simulink model "beam_control_ic_tx"  (R2022b)
settings: Solver=FixedStepAuto  StartTime=0.0  StopTime=100e-7  RelTol=1e-3
values from neighbouring files (symbols this model uses):
  beam_former_gain_array = [1 1]    [beam_control_ic_tx_parameter.m]
  Bias = 0    [ModelingRFSystemsWithAntennaArraysUsingAntennaBlockExample.m]    (also in beam_control_ic_rx_parameter.m)
  filter_gain0_0 = 0    [ModelingRFSystemsWithAntennaArraysUsingAntennaBlockExample.m]    (also in beam_control_ic_rx_parameter.m)
  filter_gain0_1 = 1/6    (= 0.166666666667)    [ModelingRFSystemsWithAntennaArraysUsingAntennaBlockExample.m]    (also in beam_control_ic_rx_parameter.m)
  filter_gain0_2 = 2/3    (= 0.666666666667)    [ModelingRFSystemsWithAntennaArraysUsingAntennaBlockExample.m]    (also in beam_control_ic_rx_parameter.m)
  filter_gain0_3 = 1/6    (= 0.166666666667)    [ModelingRFSystemsWithAntennaArraysUsingAntennaBlockExample.m]    (also in beam_control_ic_rx_parameter.m)
  filter_gain1_0 = 0    [ModelingRFSystemsWithAntennaArraysUsingAntennaBlockExample.m]    (also in beam_control_ic_rx_parameter.m)
  filter_gain1_1 = 1/2    (= 0.5)    [ModelingRFSystemsWithAntennaArraysUsingAntennaBlockExample.m]    (also in beam_control_ic_rx_parameter.m)
  filter_gain1_2 = 0    [ModelingRFSystemsWithAntennaArraysUsingAntennaBlockExample.m]    (also in beam_control_ic_rx_parameter.m)
  filter_gain1_3 = -1/2    (= -0.5)    [ModelingRFSystemsWithAntennaArraysUsingAntennaBlockExample.m]    (also in beam_control_ic_rx_parameter.m)
  filter_gain2_0 = 0    [ModelingRFSystemsWithAntennaArraysUsingAntennaBlockExample.m]    (also in beam_control_ic_rx_parameter.m)
  filter_gain2_1 = 1/2    (= 0.5)    [ModelingRFSystemsWithAntennaArraysUsingAntennaBlockExample.m]    (also in beam_control_ic_rx_parameter.m)
  filter_gain2_2 = -1    [ModelingRFSystemsWithAntennaArraysUsingAntennaBlockExample.m]    (also in beam_control_ic_rx_parameter.m)
  filter_gain2_3 = 1/2    (= 0.5)    [ModelingRFSystemsWithAntennaArraysUsingAntennaBlockExample.m]    (also in beam_control_ic_rx_parameter.m)
  filter_gain3_0 = 1/6    (= 0.166666666667)    [ModelingRFSystemsWithAntennaArraysUsingAntennaBlockExample.m]    (also in beam_control_ic_rx_parameter.m)
  filter_gain3_1 = -1/2    (= -0.5)    [ModelingRFSystemsWithAntennaArraysUsingAntennaBlockExample.m]    (also in beam_control_ic_rx_parameter.m)
  filter_gain3_2 = 1/2    (= 0.5)    [ModelingRFSystemsWithAntennaArraysUsingAntennaBlockExample.m]    (also in beam_control_ic_rx_parameter.m)
  filter_gain3_3 = -1/6    (= -0.166666666667)    [ModelingRFSystemsWithAntennaArraysUsingAntennaBlockExample.m]    (also in beam_control_ic_rx_parameter.m)
  fraction_delay = 1.5    [ModelingRFSystemsWithAntennaArraysUsingAntennaBlockExample.m]    (also in beam_control_ic_rx_parameter.m = 1)
  integer_delay = 0    [ModelingRFSystemsWithAntennaArraysUsingAntennaBlockExample.m]    (also in beam_control_ic_rx_parameter.m)
  N = 10    [ModelingRFSystemsWithAntennaArraysUsingAntennaBlockExample.m]    (also in beam_control_ic_rx_parameter.m)
  Ref = 2.048    [ModelingRFSystemsWithAntennaArraysUsingAntennaBlockExample.m]    (also in beam_control_ic_rx_parameter.m)
undefined symbols (not defined in the file or in its folder): fdesignblkfcn, gcbh, pskmod
libraries: dspsigops x5, simulink_extras x2, msbDacArchitectures x2, dspmlti4 x2, commrfcorlib x2, commeq3 x2
(part 1 of 2)
settings Model: Creator=BOBO  LastModifiedBy=BOBO

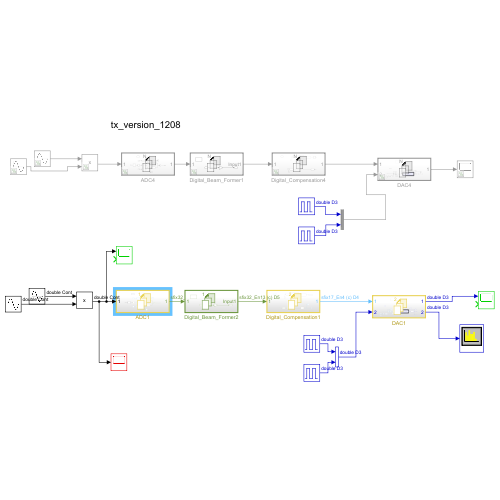
[thumbnail: Simulink's stored preview of the top-level diagram]
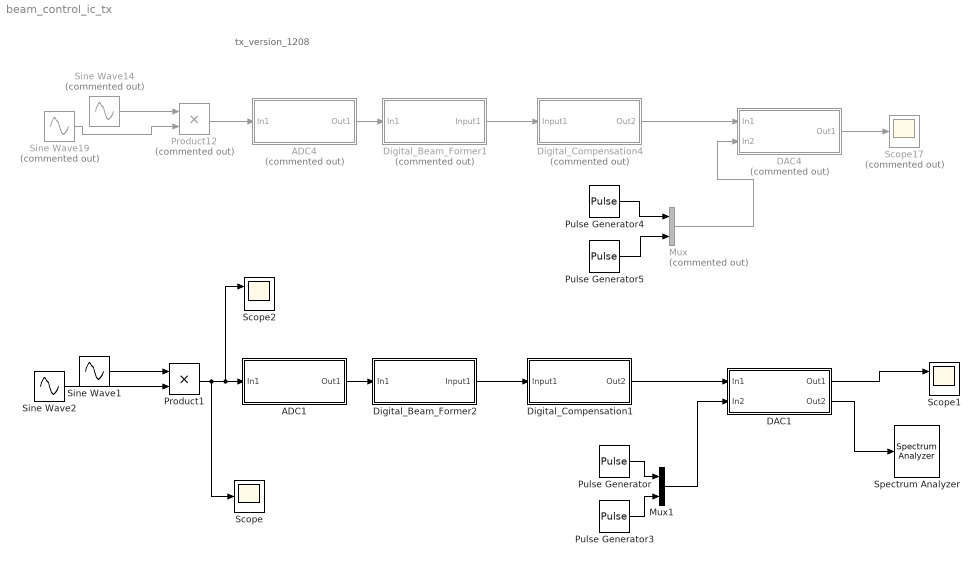
== system beam_control_ic_tx ==
  note: tx_version_1208
  ADC1 : Subsystem  TreatAsAtomicUnit=on
  ADC4 : Subsystem  Commented=on  TreatAsAtomicUnit=on
  DAC1 : Subsystem  TreatAsAtomicUnit=on
  DAC4 : Subsystem  Commented=on  TreatAsAtomicUnit=on
  Digital_Beam_Former1 : Subsystem  Commented=on  TreatAsAtomicUnit=on
  Digital_Beam_Former2 : Subsystem  TreatAsAtomicUnit=on
  Digital_Compensation1 : Subsystem  TreatAsAtomicUnit=on
  Digital_Compensation4 : Subsystem  Commented=on  TreatAsAtomicUnit=on
  Mux : Mux  Commented=on  Inputs=2
  Mux1 : Mux  Inputs=2
  Product1 : Product
  Product12 : Product  Commented=on
  Pulse Generator{,3..5} (4 alike) : DiscretePulseGenerator  PulseType=Time based  Period=1e-9  PulseWidth=50
  Scope : Scope
  Scope1 : Scope  NumInputPorts=2
  Scope17 : Scope  Commented=on
  Scope2 : Scope  NumInputPorts=2
  Sine Wave1 : Sin  Frequency=2*pi*3.25e9  SampleTime=0
  Sine Wave14 : Sin  Commented=on  Frequency=2*pi*3.25e9  SampleTime=0
  Sine Wave19 : Sin  Commented=on  Frequency=2*pi*62.5e6  SampleTime=0
  Sine Wave2 : Sin  Frequency=2*pi*62.5e6  SampleTime=0
  Spectrum Analyzer : SpectrumAnalyzer
  wires:
  Digital_Compensation4/1(Out2) -> DAC4/1(In1)
  ADC4/1(Out1) -> Digital_Beam_Former1/1(In1)
  Sine Wave14/1 -> Product12/1
  Sine Wave19/1 -> Product12/2
  Product12/1 -> ADC4/1(In1)
  DAC4/1(Out1) -> Scope17/1
  Digital_Beam_Former1/1(Input1) -> Digital_Compensation4/1(Input1)
  Pulse Generator4/1 -> Mux/1
  Pulse Generator5/1 -> Mux/2
  Mux/1 -> DAC4/2(In2)
  Mux1/1 -> DAC1/2(In2)
  Pulse Generator3/1 -> Mux1/2
  Pulse Generator/1 -> Mux1/1
  Digital_Beam_Former2/1(Input1) -> Digital_Compensation1/1(Input1)
  Product1/1 -> Scope/1, Scope2/1, ADC1/1(In1)
  Sine Wave2/1 -> Product1/2
  Sine Wave1/1 -> Product1/1
  ADC1/1(Out1) -> Digital_Beam_Former2/1(In1)
  Digital_Compensation1/1(Out2) -> DAC1/1(In1)
  DAC1/2(Out2) -> Spectrum Analyzer/1
  DAC1/1(Out1) -> Scope1/1

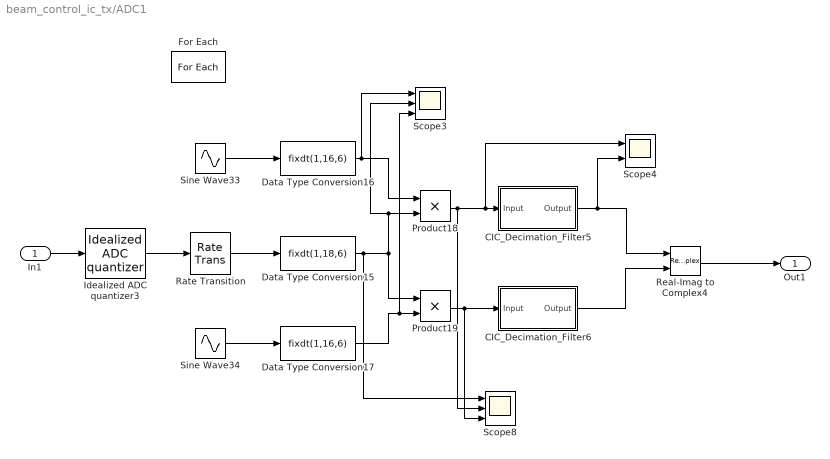
== system beam_control_ic_tx/ADC1 ==
  In1 : Inport  Partition=on  PartitionDimension=1  PartitionWidth=1  PartitionOffset=0
  CIC_Decimation_Filter5 : Subsystem  Tag=FilterWizardSubSystem
      settings: ErrorFcn=dspFilterRealizedInBasicElemsAlgLoopErrFcnCallback
  CIC_Decimation_Filter6 : Subsystem  Tag=FilterWizardSubSystem
      settings: ErrorFcn=dspFilterRealizedInBasicElemsAlgLoopErrFcnCallback
  Data Type Conversion15 : DataTypeConversion  OutDataTypeStr=fixdt(1,18,6)  SaturateOnIntegerOverflow=off  RndMeth=Floor
  Data Type Conversion16 : DataTypeConversion  OutDataTypeStr=fixdt(1,16,6)  SaturateOnIntegerOverflow=off  RndMeth=Floor
  Data Type Conversion17 : DataTypeConversion  OutDataTypeStr=fixdt(1,16,6)  SaturateOnIntegerOverflow=off  RndMeth=Floor
  For Each : ForEach  DisableCoverage=on
  Idealized ADC quantizer3 : simulink_extras/Additional Discrete/Idealized ADC quantizer  NumberOfConverterBits=8  Vmin=-1  Vmax=1  OutputDataType=double  OutputNegativeValues=on
  Product18 : Product
  Product19 : Product
  Rate Transition : RateTransition  OutPortSampleTime=1/1e9
  Real-Imag to Complex4 : RealImagToComplex
  Scope3 : Scope  NumInputPorts=3
  Scope4 : Scope  NumInputPorts=2
  Scope8 : Scope  NumInputPorts=3
  Sine Wave33 : Sin  Frequency=2*pi*250e6  Phase=1.57  SampleTime=1/1e9
  Sine Wave34 : Sin  Frequency=2*pi*250e6  SampleTime=1/1e9
  Out1 : Outport  ConcatenationDimension=1
  wires:
  CIC_Decimation_Filter6/1(Output) -> Real-Imag to Complex4/2
  Sine Wave33/1 -> Data Type Conversion16/1
  Product19/1 -> CIC_Decimation_Filter6/1(Input), Scope8/3
  Data Type Conversion16/1 -> Scope3/1, Product18/1
  Sine Wave34/1 -> Data Type Conversion17/1
  Data Type Conversion17/1 -> Product19/2, Scope3/3
  Real-Imag to Complex4/1 -> Out1/1
  In1/1 -> Idealized ADC quantizer3/1
  Rate Transition/1 -> Data Type Conversion15/1
  Idealized ADC quantizer3/1 -> Rate Transition/1
  Data Type Conversion15/1 -> Scope3/2, Product18/2, Product19/1, Scope8/1
  Product18/1 -> Scope8/2, CIC_Decimation_Filter5/1(Input), Scope4/1
  CIC_Decimation_Filter5/1(Output) -> Real-Imag to Complex4/1, Scope4/2

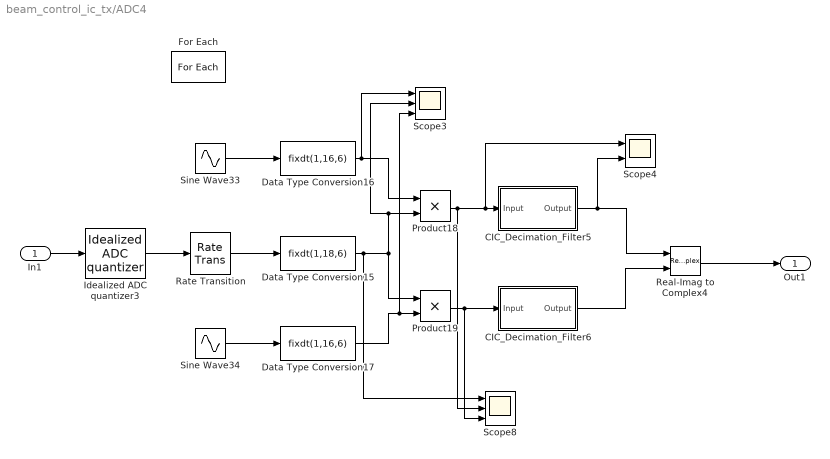
== system beam_control_ic_tx/ADC4 ==
  In1 : Inport  Partition=on  PartitionDimension=1  PartitionWidth=1  PartitionOffset=0
  CIC_Decimation_Filter5 : Subsystem  Tag=FilterWizardSubSystem
      settings: ErrorFcn=dspFilterRealizedInBasicElemsAlgLoopErrFcnCallback
  CIC_Decimation_Filter6 : Subsystem  Tag=FilterWizardSubSystem
      settings: ErrorFcn=dspFilterRealizedInBasicElemsAlgLoopErrFcnCallback
  Data Type Conversion15 : DataTypeConversion  OutDataTypeStr=fixdt(1,18,6)  SaturateOnIntegerOverflow=off  RndMeth=Floor
  Data Type Conversion16 : DataTypeConversion  OutDataTypeStr=fixdt(1,16,6)  SaturateOnIntegerOverflow=off  RndMeth=Floor
  Data Type Conversion17 : DataTypeConversion  OutDataTypeStr=fixdt(1,16,6)  SaturateOnIntegerOverflow=off  RndMeth=Floor
  For Each : ForEach  DisableCoverage=on
  Idealized ADC quantizer3 : simulink_extras/Additional Discrete/Idealized ADC quantizer  NumberOfConverterBits=12  Vmin=-1  Vmax=1  OutputDataType=double  OutputNegativeValues=on
  Product18 : Product
  Product19 : Product
  Rate Transition : RateTransition  OutPortSampleTime=1/1e9
  Real-Imag to Complex4 : RealImagToComplex
  Scope3 : Scope  NumInputPorts=3
  Scope4 : Scope  NumInputPorts=2
  Scope8 : Scope  NumInputPorts=3
  Sine Wave33 : Sin  Frequency=2*pi*250e6  Phase=1.57  SampleTime=1/1e9
  Sine Wave34 : Sin  Frequency=2*pi*250e6  SampleTime=1/1e9
  Out1 : Outport  ConcatenationDimension=1
  wires:
  CIC_Decimation_Filter5/1(Output) -> Scope4/2, Real-Imag to Complex4/1
  Product18/1 -> Scope4/1, CIC_Decimation_Filter5/1(Input), Scope8/2
  Data Type Conversion15/1 -> Scope8/1, Product19/1, Product18/2, Scope3/2
  Idealized ADC quantizer3/1 -> Rate Transition/1
  Rate Transition/1 -> Data Type Conversion15/1
  In1/1 -> Idealized ADC quantizer3/1
  Real-Imag to Complex4/1 -> Out1/1
  Data Type Conversion17/1 -> Scope3/3, Product19/2
  Sine Wave34/1 -> Data Type Conversion17/1
  Data Type Conversion16/1 -> Product18/1, Scope3/1
  Product19/1 -> Scope8/3, CIC_Decimation_Filter6/1(Input)
  Sine Wave33/1 -> Data Type Conversion16/1
  CIC_Decimation_Filter6/1(Output) -> Real-Imag to Complex4/2

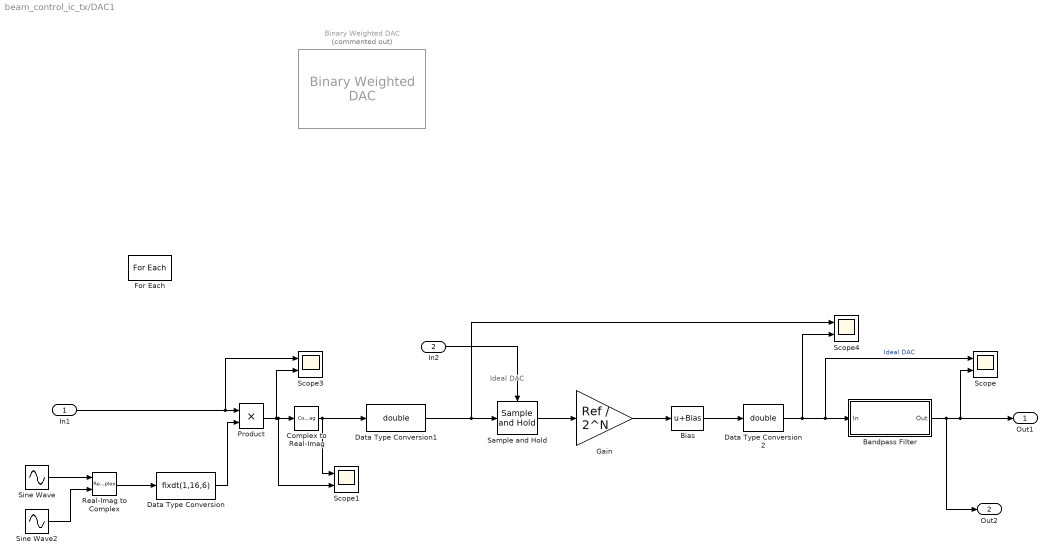
== system beam_control_ic_tx/DAC1 ==
  note: Ideal DAC
  In1 : Inport  Partition=on  PartitionDimension=1  PartitionWidth=1  PartitionOffset=0
  In2 : Inport  Port=2  Partition=on  PartitionDimension=1  PartitionWidth=1  PartitionOffset=0
  Bandpass Filter : Subsystem  DialogController=fdesignblkfcn  InitFcn=fdesignblkfcn(gcbh, {'InitFcn'});  mask(Bandpass Filter){}
      mask help: Design a bandpass filter
      settings: CopyFcn=fdesignblkfcn(gcbh, {'CopyFcn'});
      mask Help: helpview(mapfilelocation('dsp'), 'dspbandpassfilter');
      mask Display: disp('Bandpass');
  Bias : Bias  Bias=Bias  SaturateOnIntegerOverflow=off
  Binary Weighted DAC : msbDacArchitectures/Binary Weighted DAC  Commented=on  NBits=5  Polarity=Bipolar  ExtStartClk=on  StartFreq=1e6  Ref=2  Bias=0  ReadySignal=off  EnableLinearityImpairments=on  OffsetError=0  OffsetErrorUnit=LSB  GainError=0  GainErrorUnit=LSB  EnableTimingImpairments=on  TimingSpecification=Settling time  SettlingTime=2e-7  SettlingTimeTolerance=0.5  RisingSlewRate=5015625  FallingSlewRate=-5015625
  Complex to Real-Imag : ComplexToRealImag  Output=Real
  Data Type Conversion : DataTypeConversion  OutDataTypeStr=fixdt(1,16,6)  SaturateOnIntegerOverflow=off  RndMeth=Floor
  Data Type Conversion1 : DataTypeConversion  OutDataTypeStr=double  SaturateOnIntegerOverflow=off  RndMeth=Floor
  Data Type Conversion2 : DataTypeConversion  OutDataTypeStr=double  SaturateOnIntegerOverflow=off  RndMeth=Floor
  For Each : ForEach  DisableCoverage=on
  Gain : Gain  Gain=Ref / 2^N
  Product : Product
  Real-Imag to Complex : RealImagToComplex
  Sample and Hold : dspsigops/Sample and Hold  trig=Rising edge  initCond=0  latchinput=off
  Scope{,1,3..4} (4 alike) : Scope  NumInputPorts=2
  Sine Wave : Sin  Frequency=2*pi*250e6  Phase=1.57  SampleTime=1/1e9
  Sine Wave2 : Sin  Frequency=2*pi*250e6  SampleTime=1/1e9
  Out1 : Outport  ConcatenationDimension=1
  Out2 : Outport  Port=2  ConcatenationDimension=1
  wires:
  Bandpass Filter/1(Out) -> Out2/1, Out1/1, Scope/2
  In2/1 -> Sample and Hold/Trigger
  Sample and Hold/1 -> Gain/1
  Gain/1 -> Bias/1
  Bias/1 -> Data Type Conversion2/1
  Data Type Conversion1/1 -> Sample and Hold/1, Scope4/1
  Data Type Conversion2/1 -> Bandpass Filter/1(In), Scope/1, Scope4/2  "Ideal DAC"
  Real-Imag to Complex/1 -> Data Type Conversion/1
  Sine Wave2/1 -> Real-Imag to Complex/2
  Sine Wave/1 -> Real-Imag to Complex/1
  In1/1 -> Scope3/1, Product/1
  Product/1 -> Scope3/2, Complex to Real-Imag/1, Scope1/2
  Complex to Real-Imag/1 -> Scope1/1, Data Type Conversion1/1
  Data Type Conversion/1 -> Product/2

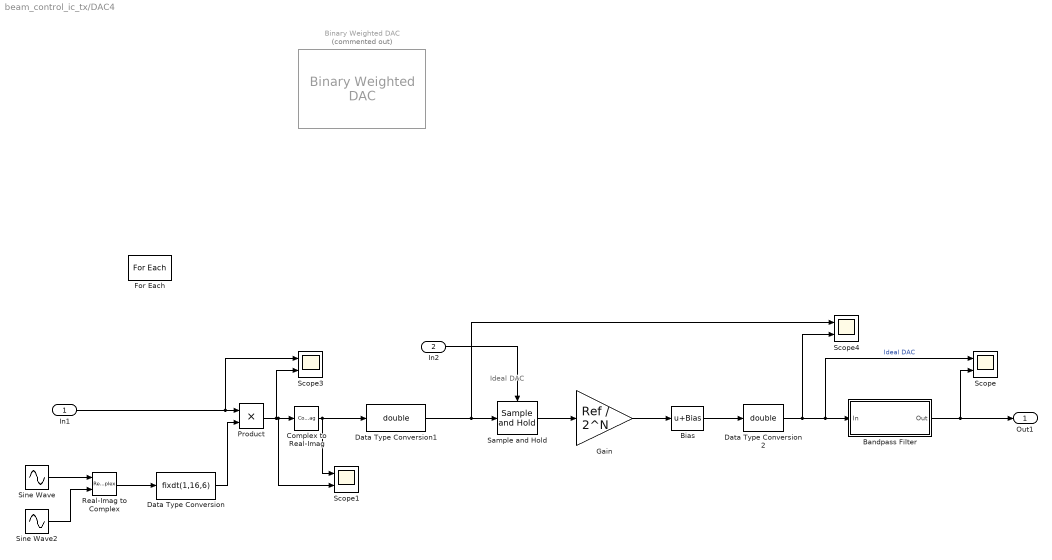
== system beam_control_ic_tx/DAC4 ==
  note: Ideal DAC
  In1 : Inport  Partition=on  PartitionDimension=1  PartitionWidth=1  PartitionOffset=0
  In2 : Inport  Port=2  Partition=on  PartitionDimension=1  PartitionWidth=1  PartitionOffset=0
  Bandpass Filter : Subsystem  DialogController=fdesignblkfcn  InitFcn=fdesignblkfcn(gcbh, {'InitFcn'});  mask(Bandpass Filter){}
      mask help: Design a bandpass filter
      settings: CopyFcn=fdesignblkfcn(gcbh, {'CopyFcn'});
      mask Help: helpview(mapfilelocation('dsp'), 'dspbandpassfilter');
      mask Display: disp('Bandpass');
  Bias : Bias  Bias=Bias  SaturateOnIntegerOverflow=off
  Binary Weighted DAC : msbDacArchitectures/Binary Weighted DAC  Commented=on  NBits=5  Polarity=Bipolar  ExtStartClk=on  StartFreq=1e6  Ref=2  Bias=0  ReadySignal=off  EnableLinearityImpairments=on  OffsetError=0  OffsetErrorUnit=LSB  GainError=0  GainErrorUnit=LSB  EnableTimingImpairments=on  TimingSpecification=Settling time  SettlingTime=2e-7  SettlingTimeTolerance=0.5  RisingSlewRate=5015625  FallingSlewRate=-5015625
  Complex to Real-Imag : ComplexToRealImag  Output=Real
  Data Type Conversion : DataTypeConversion  OutDataTypeStr=fixdt(1,16,6)  SaturateOnIntegerOverflow=off  RndMeth=Floor
  Data Type Conversion1 : DataTypeConversion  OutDataTypeStr=double  SaturateOnIntegerOverflow=off  RndMeth=Floor
  Data Type Conversion2 : DataTypeConversion  OutDataTypeStr=double  SaturateOnIntegerOverflow=off  RndMeth=Floor
  For Each : ForEach  DisableCoverage=on
  Gain : Gain  Gain=Ref / 2^N
  Product : Product
  Real-Imag to Complex : RealImagToComplex
  Sample and Hold : dspsigops/Sample and Hold  trig=Rising edge  initCond=0  latchinput=off
  Scope{,1,3..4} (4 alike) : Scope  NumInputPorts=2
  Sine Wave : Sin  Frequency=2*pi*250e6  Phase=1.57  SampleTime=1/1e9
  Sine Wave2 : Sin  Frequency=2*pi*250e6  SampleTime=1/1e9
  Out1 : Outport  ConcatenationDimension=1
  wires:
  Data Type Conversion/1 -> Product/2
  Complex to Real-Imag/1 -> Data Type Conversion1/1, Scope1/1
  Product/1 -> Scope1/2, Complex to Real-Imag/1, Scope3/2
  In1/1 -> Product/1, Scope3/1
  Sine Wave/1 -> Real-Imag to Complex/1
  Sine Wave2/1 -> Real-Imag to Complex/2
  Real-Imag to Complex/1 -> Data Type Conversion/1
  Data Type Conversion2/1 -> Scope4/2, Scope/1, Bandpass Filter/1(In)  "Ideal DAC"
  Data Type Conversion1/1 -> Scope4/1, Sample and Hold/1
  Bias/1 -> Data Type Conversion2/1
  Gain/1 -> Bias/1
  Sample and Hold/1 -> Gain/1
  In2/1 -> Sample and Hold/Trigger
  Bandpass Filter/1(Out) -> Scope/2, Out1/1

== system beam_control_ic_tx/Digital_Beam_Former1 ==
  In1 : Inport  Partition=on  PartitionDimension=1  PartitionWidth=1  PartitionOffset=0
  For Each : ForEach  DisableCoverage=on
  Gain : Gain  Gain=beam_former_gain_array  OutDataTypeStr=fixdt(1,32,13)
  Input1 : Outport  ConcatenationDimension=1
  wires:
  In1/1 -> Gain/1
  Gain/1 -> Input1/1

== system beam_control_ic_tx/Digital_Beam_Former2 ==
  In1 : Inport  Partition=on  PartitionDimension=1  PartitionWidth=1  PartitionOffset=0
  For Each : ForEach  DisableCoverage=on
  Gain : Gain  Gain=beam_former_gain_array  OutDataTypeStr=fixdt(1,32,13)
  Input1 : Outport  ConcatenationDimension=1
  wires:
  Gain/1 -> Input1/1
  In1/1 -> Gain/1

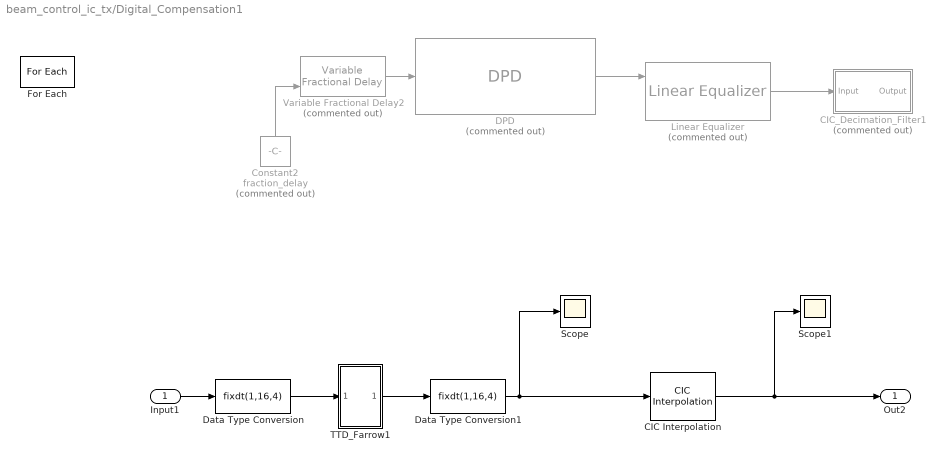
== system beam_control_ic_tx/Digital_Compensation1 ==
  Input1 : Inport  Partition=on  PartitionDimension=1  PartitionWidth=1  PartitionOffset=0
  CIC Interpolation : dspmlti4/CIC Interpolation  filtFrom=Dialog parameters  filtobj=Hm_interp  ftype=Interpolator  R=2  M=1  N=2  filterInternals=Full precision  BPS=[16 16 16 16]  FLPS=0  outputWordLength=32  outputFracLength=0  launchFVT=off  framing=Allow multirate processing  OutputFrames=off
      settings: LibrarySourceBlock=|
      | dsphdlsupportfiltering/CIC
      | Interpolation
  CIC_Decimation_Filter1 : Subsystem  Tag=FilterWizardSubSystem  Commented=on
      settings: ErrorFcn=dspFilterRealizedInBasicElemsAlgLoopErrFcnCallback
  Constant2 : Constant  Commented=on  Value=fraction_delay  OutDataTypeStr=fixdt(1,16,6)
  DPD : commrfcorlib/DPD  Commented=on  PolynomialType=Memory polynomial  CoefficientSource=Property  Coefficients=complex([1 0 0 0 0; 0 0 0 0 0; 0 0 0 0 0])  SimulateUsing=Code generation
  Data Type Conversion : DataTypeConversion  OutDataTypeStr=fixdt(1,16,4)  SaturateOnIntegerOverflow=off  RndMeth=Floor
  Data Type Conversion1 : DataTypeConversion  OutDataTypeStr=fixdt(1,16,4)  SaturateOnIntegerOverflow=off  RndMeth=Floor
  For Each : ForEach  DisableCoverage=on
  Linear Equalizer : commeq3/Linear Equalizer  Commented=on  NumTaps=5  Constellation=pskmod( 0:3, 4, pi/4, 'bin' )  InputSamplesPerSymbol=1  Algorithm=LMS  StepSize=0.01  ForgettingFactor=0.99  InitialInverseCorrelationMatrix=0.1  ReferenceTap=3  InputDelay=0  AdaptWeightsSource=Property  AdaptWeights=on  InitialWeightsSource=Auto  InitialWeights=0  TrainingInitialWeights=0  BlindInitialWeights=[ 0; 0; 1; 0; 0 ]  WeightUpdatePeriod=1  TrainingFlagInputPort=off  AdaptAfterTraining=on  ResetInputPort=off  ErrorOutputPort=off  TapWeightsOutputPort=off  SimulateUsing=Code generation
  Scope : Scope
  Scope1 : Scope
  TTD_Farrow1 : Subsystem
  Variable Fractional Delay2 : dspsigops/Variable Fractional Delay  Commented=on  mode=OBSOLETE  modeActive=Linear  L=4  FarrowL=4  R=10  alpha=1  dmax=100  InputProcessing=Columns as channels (frame based)  ic=0  noDFT=off  fallbackFIR=Clip to the minimum value necessary for centered kernel  fallbackFarrow=Clip to the minimum value necessary for centered kernel  roundingMode=Zero  overflowMode=off
  Out2 : Outport  ConcatenationDimension=1
  wires:
  CIC Interpolation/1 -> Scope1/1, Out2/1
  Linear Equalizer/1 -> CIC_Decimation_Filter1/1(Input)
  DPD/1 -> Linear Equalizer/1
  Variable Fractional Delay2/1 -> DPD/1
  Constant2/1 -> Variable Fractional Delay2/2
  Input1/1 -> Data Type Conversion/1
  TTD_Farrow1/1(Output) -> Data Type Conversion1/1
  Data Type Conversion/1 -> TTD_Farrow1/1(In1)
  Data Type Conversion1/1 -> CIC Interpolation/1, Scope/1

== system beam_control_ic_tx/Digital_Compensation4 ==
  Input1 : Inport  Partition=on  PartitionDimension=1  PartitionWidth=1  PartitionOffset=0
  CIC Interpolation : dspmlti4/CIC Interpolation  filtFrom=Dialog parameters  filtobj=Hm_interp  ftype=Interpolator  R=2  M=1  N=2  filterInternals=Full precision  BPS=[16 16 16 16]  FLPS=0  outputWordLength=32  outputFracLength=0  launchFVT=off  framing=Allow multirate processing  OutputFrames=off
      settings: LibrarySourceBlock=|
      | dsphdlsupportfiltering/CIC
      | Interpolation
  CIC_Decimation_Filter3 : Subsystem  Tag=FilterWizardSubSystem
      settings: ErrorFcn=dspFilterRealizedInBasicElemsAlgLoopErrFcnCallback
  Constant1 : Constant  Value=fraction_delay  OutDataTypeStr=fixdt(1,16,6)
  Constant2 : Constant  Commented=on  Value=fraction_delay  OutDataTypeStr=fixdt(1,16,6)
  DPD : commrfcorlib/DPD  Commented=on  PolynomialType=Memory polynomial  CoefficientSource=Property  Coefficients=complex([1 0 0 0 0; 0 0 0 0 0; 0 0 0 0 0])  SimulateUsing=Code generation
  For Each : ForEach  DisableCoverage=on
  Linear Equalizer : commeq3/Linear Equalizer  Commented=on  NumTaps=5  Constellation=pskmod( 0:3, 4, pi/4, 'bin' )  InputSamplesPerSymbol=1  Algorithm=LMS  StepSize=0.01  ForgettingFactor=0.99  InitialInverseCorrelationMatrix=0.1  ReferenceTap=3  InputDelay=0  AdaptWeightsSource=Property  AdaptWeights=on  InitialWeightsSource=Auto  InitialWeights=0  TrainingInitialWeights=0  BlindInitialWeights=[ 0; 0; 1; 0; 0 ]  WeightUpdatePeriod=1  TrainingFlagInputPort=off  AdaptAfterTraining=on  ResetInputPort=off  ErrorOutputPort=off  TapWeightsOutputPort=off  SimulateUsing=Code generation
  Variable Fractional Delay1 : dspsigops/Variable Fractional Delay  mode=OBSOLETE  modeActive=Linear  L=4  FarrowL=4  R=10  alpha=1  dmax=100  InputProcessing=Columns as channels (frame based)  ic=0  noDFT=off  fallbackFIR=Clip to the minimum value necessary for centered kernel  fallbackFarrow=Clip to the minimum value necessary for centered kernel  roundingMode=Zero  overflowMode=off
  Variable Fractional Delay2 : dspsigops/Variable Fractional Delay  Commented=on  mode=OBSOLETE  modeActive=Linear  L=4  FarrowL=4  R=10  alpha=1  dmax=100  InputProcessing=Columns as channels (frame based)  ic=0  noDFT=off  fallbackFIR=Clip to the minimum value necessary for centered kernel  fallbackFarrow=Clip to the minimum value necessary for centered kernel  roundingMode=Zero  overflowMode=off
  Out2 : Outport  ConcatenationDimension=1
  wires:
  Variable Fractional Delay1/1 -> CIC_Decimation_Filter3/1(Input)
  Constant1/1 -> Variable Fractional Delay1/2
  Constant2/1 -> Variable Fractional Delay2/2
  Variable Fractional Delay2/1 -> DPD/1
  DPD/1 -> Linear Equalizer/1
  Linear Equalizer/1 -> CIC Interpolation/1
  CIC_Decimation_Filter3/1(Output) -> Out2/1
  Input1/1 -> Variable Fractional Delay1/1

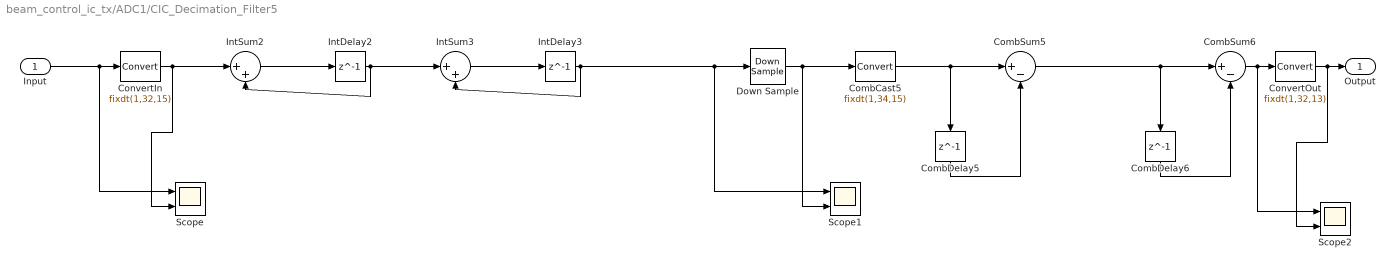
== system beam_control_ic_tx/ADC1/CIC_Decimation_Filter5 ==
  Input : Inport
  CombCast5 : DataTypeConversion  OutDataTypeStr=fixdt(1,34,15)  SaturateOnIntegerOverflow=off  RndMeth=Floor
  CombDelay5 : Delay  DelayLength=1  InitialCondition=0
  CombDelay6 : Delay  DelayLength=1  InitialCondition=0
  CombSum5 : Sum  Inputs=|+-  AccumDataTypeStr=fixdt(1,34,15)  OutDataTypeStr=fixdt(1,34,15)
  CombSum6 : Sum  Inputs=|+-  AccumDataTypeStr=fixdt(1,34,15)  OutDataTypeStr=fixdt(1,34,15)
  ConvertIn : DataTypeConversion  OutDataTypeStr=fixdt(1,32,15)  RndMeth=Nearest
  ConvertOut : DataTypeConversion  OutDataTypeStr=fixdt(1,32,13)  SaturateOnIntegerOverflow=off  RndMeth=Floor
  Down Sample : DownSample  RateOptions=Allow multirate processing  AllowArbitraryFixedInput=on
  IntDelay2 : Delay  DelayLength=1  InitialCondition=0
  IntDelay3 : Delay  DelayLength=1  InitialCondition=0
  IntSum2 : Sum  Inputs=|++  AccumDataTypeStr=fixdt(1,34,15)  OutDataTypeStr=fixdt(1,34,15)
  IntSum3 : Sum  Inputs=|++  AccumDataTypeStr=fixdt(1,34,15)  OutDataTypeStr=fixdt(1,34,15)
  Scope : Scope  NumInputPorts=2
  Scope1 : Scope  NumInputPorts=2
  Scope2 : Scope  NumInputPorts=2
  Output : Outport
  wires:
  ConvertOut/1 -> Output/1, Scope2/2
  CombDelay6/1 -> CombSum6/2
  CombSum6/1 -> ConvertOut/1, Scope2/1
  CombCast5/1 -> CombDelay5/1, CombSum5/1
  CombDelay5/1 -> CombSum5/2
  CombSum5/1 -> CombDelay6/1, CombSum6/1
  Down Sample/1 -> CombCast5/1, Scope1/2
  IntDelay3/1 -> Down Sample/1, Scope1/1, IntSum3/2
  IntSum3/1 -> IntDelay3/1
  IntDelay2/1 -> IntSum3/1, IntSum2/2
  IntSum2/1 -> IntDelay2/1
  ConvertIn/1 -> IntSum2/1, Scope/2
  Input/1 -> ConvertIn/1, Scope/1

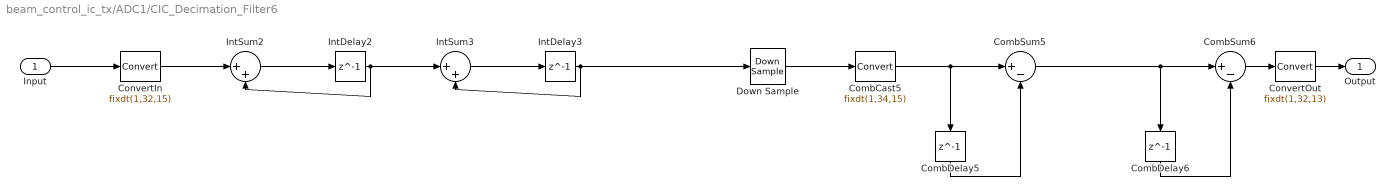
== system beam_control_ic_tx/ADC1/CIC_Decimation_Filter6 ==
  Input : Inport
  CombCast5 : DataTypeConversion  OutDataTypeStr=fixdt(1,34,15)  SaturateOnIntegerOverflow=off  RndMeth=Floor
  CombDelay5 : Delay  DelayLength=1  InitialCondition=0
  CombDelay6 : Delay  DelayLength=1  InitialCondition=0
  CombSum5 : Sum  Inputs=|+-  AccumDataTypeStr=fixdt(1,34,15)  OutDataTypeStr=fixdt(1,34,15)
  CombSum6 : Sum  Inputs=|+-  AccumDataTypeStr=fixdt(1,34,15)  OutDataTypeStr=fixdt(1,34,15)
  ConvertIn : DataTypeConversion  OutDataTypeStr=fixdt(1,32,15)  RndMeth=Nearest
  ConvertOut : DataTypeConversion  OutDataTypeStr=fixdt(1,32,13)  SaturateOnIntegerOverflow=off  RndMeth=Floor
  Down Sample : DownSample  RateOptions=Allow multirate processing  AllowArbitraryFixedInput=on
  IntDelay2 : Delay  DelayLength=1  InitialCondition=0
  IntDelay3 : Delay  DelayLength=1  InitialCondition=0
  IntSum2 : Sum  Inputs=|++  AccumDataTypeStr=fixdt(1,34,15)  OutDataTypeStr=fixdt(1,34,15)
  IntSum3 : Sum  Inputs=|++  AccumDataTypeStr=fixdt(1,34,15)  OutDataTypeStr=fixdt(1,34,15)
  Output : Outport
  wires:
  Input/1 -> ConvertIn/1
  ConvertIn/1 -> IntSum2/1
  IntSum2/1 -> IntDelay2/1
  IntDelay2/1 -> IntSum2/2, IntSum3/1
  IntSum3/1 -> IntDelay3/1
  IntDelay3/1 -> IntSum3/2, Down Sample/1
  Down Sample/1 -> CombCast5/1
  CombSum5/1 -> CombSum6/1, CombDelay6/1
  CombDelay5/1 -> CombSum5/2
  CombCast5/1 -> CombSum5/1, CombDelay5/1
  CombSum6/1 -> ConvertOut/1
  CombDelay6/1 -> CombSum6/2
  ConvertOut/1 -> Output/1

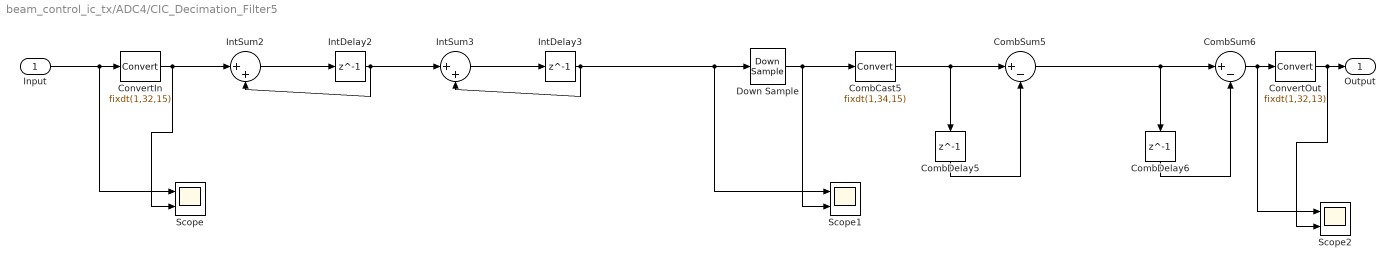
== system beam_control_ic_tx/ADC4/CIC_Decimation_Filter5 ==
  Input : Inport
  CombCast5 : DataTypeConversion  OutDataTypeStr=fixdt(1,34,15)  SaturateOnIntegerOverflow=off  RndMeth=Floor
  CombDelay5 : Delay  DelayLength=1  InitialCondition=0
  CombDelay6 : Delay  DelayLength=1  InitialCondition=0
  CombSum5 : Sum  Inputs=|+-  AccumDataTypeStr=fixdt(1,34,15)  OutDataTypeStr=fixdt(1,34,15)
  CombSum6 : Sum  Inputs=|+-  AccumDataTypeStr=fixdt(1,34,15)  OutDataTypeStr=fixdt(1,34,15)
  ConvertIn : DataTypeConversion  OutDataTypeStr=fixdt(1,32,15)  RndMeth=Nearest
  ConvertOut : DataTypeConversion  OutDataTypeStr=fixdt(1,32,13)  SaturateOnIntegerOverflow=off  RndMeth=Floor
  Down Sample : DownSample  RateOptions=Allow multirate processing  AllowArbitraryFixedInput=on
  IntDelay2 : Delay  DelayLength=1  InitialCondition=0
  IntDelay3 : Delay  DelayLength=1  InitialCondition=0
  IntSum2 : Sum  Inputs=|++  AccumDataTypeStr=fixdt(1,34,15)  OutDataTypeStr=fixdt(1,34,15)
  IntSum3 : Sum  Inputs=|++  AccumDataTypeStr=fixdt(1,34,15)  OutDataTypeStr=fixdt(1,34,15)
  Scope : Scope  NumInputPorts=2
  Scope1 : Scope  NumInputPorts=2
  Scope2 : Scope  NumInputPorts=2
  Output : Outport
  wires:
  Input/1 -> Scope/1, ConvertIn/1
  ConvertIn/1 -> Scope/2, IntSum2/1
  IntSum2/1 -> IntDelay2/1
  IntDelay2/1 -> IntSum2/2, IntSum3/1
  IntSum3/1 -> IntDelay3/1
  IntDelay3/1 -> IntSum3/2, Scope1/1, Down Sample/1
  Down Sample/1 -> Scope1/2, CombCast5/1
  CombSum5/1 -> CombSum6/1, CombDelay6/1
  CombDelay5/1 -> CombSum5/2
  CombCast5/1 -> CombSum5/1, CombDelay5/1
  CombSum6/1 -> Scope2/1, ConvertOut/1
  CombDelay6/1 -> CombSum6/2
  ConvertOut/1 -> Scope2/2, Output/1

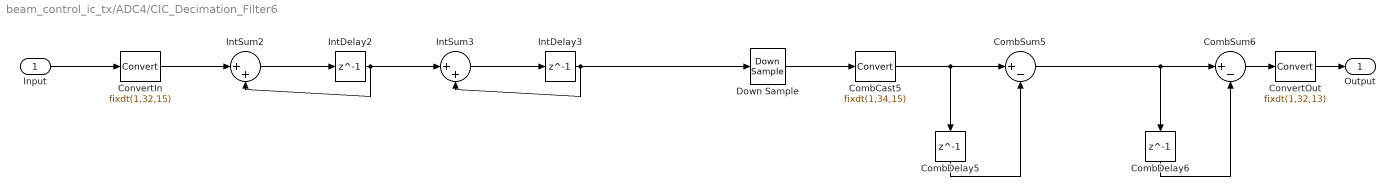
== system beam_control_ic_tx/ADC4/CIC_Decimation_Filter6 ==
  Input : Inport
  CombCast5 : DataTypeConversion  OutDataTypeStr=fixdt(1,34,15)  SaturateOnIntegerOverflow=off  RndMeth=Floor
  CombDelay5 : Delay  DelayLength=1  InitialCondition=0
  CombDelay6 : Delay  DelayLength=1  InitialCondition=0
  CombSum5 : Sum  Inputs=|+-  AccumDataTypeStr=fixdt(1,34,15)  OutDataTypeStr=fixdt(1,34,15)
  CombSum6 : Sum  Inputs=|+-  AccumDataTypeStr=fixdt(1,34,15)  OutDataTypeStr=fixdt(1,34,15)
  ConvertIn : DataTypeConversion  OutDataTypeStr=fixdt(1,32,15)  RndMeth=Nearest
  ConvertOut : DataTypeConversion  OutDataTypeStr=fixdt(1,32,13)  SaturateOnIntegerOverflow=off  RndMeth=Floor
  Down Sample : DownSample  RateOptions=Allow multirate processing  AllowArbitraryFixedInput=on
  IntDelay2 : Delay  DelayLength=1  InitialCondition=0
  IntDelay3 : Delay  DelayLength=1  InitialCondition=0
  IntSum2 : Sum  Inputs=|++  AccumDataTypeStr=fixdt(1,34,15)  OutDataTypeStr=fixdt(1,34,15)
  IntSum3 : Sum  Inputs=|++  AccumDataTypeStr=fixdt(1,34,15)  OutDataTypeStr=fixdt(1,34,15)
  Output : Outport
  wires:
  ConvertOut/1 -> Output/1
  CombDelay6/1 -> CombSum6/2
  CombSum6/1 -> ConvertOut/1
  CombCast5/1 -> CombDelay5/1, CombSum5/1
  CombDelay5/1 -> CombSum5/2
  CombSum5/1 -> CombDelay6/1, CombSum6/1
  Down Sample/1 -> CombCast5/1
  IntDelay3/1 -> Down Sample/1, IntSum3/2
  IntSum3/1 -> IntDelay3/1
  IntDelay2/1 -> IntSum3/1, IntSum2/2
  IntSum2/1 -> IntDelay2/1
  ConvertIn/1 -> IntSum2/1
  Input/1 -> ConvertIn/1

== system beam_control_ic_tx/DAC1/Bandpass Filter ==
  In : Inport
  Generated Filter Block : DiscreteFir  Tag=BlockMethodSubSystem  Coefficients=[0.000646930090822004961 -0.000497671160010674184 0.000669682907159244644 -0.000863265638125511629 0.00107434177424948476 -0.00129824676533420906 0.00152885752867004242 -0.00175777516308470768 0.00197671818651552235 -0.00217850290587446975 0.00235243304274583391 -0.00249259080896993904 0.00259084634576933412 -0.0026418349968450397 0.00264154918254561055 -0.00258837893165569585 0.00248264490979798261 -0.00232745614511145615 0.00212849245206465226 -0.00189279255657850282 0.0016304079418392875 -0.00135202124480155589 0.00106987179602428123 -0.000796462149747330372 0.000544282899543148402 -0.000324674472872522879 0.000147672218659015975 -2.12226247930935585e-05 -4.9565044166900718e-05 6.19488885635968711e-05 -1.66316267344174262e-05 -8.28963724888165387e-05 0.000230094471952851931 -0.00041595101274204821 0.000629153127361864462 -0.000857085630365267415 0.00108634009336276011 -0.00130342500304474196 0.00149591580123278889 -0.00165270678033890145 0.00176505782791396698 -0.00182687955159942933 0.0018353046261611744 -0.00179065424647863874 0.00169671308428531037 -0.00156030395279683348 0.00139089202816489177 -0.00120018052220560723 0.00100110530603660097 -0.000807263494093518608 0.000631881827906341509 -0.000487095048881364123 0.000382972539024237224 -0.000327066855091207032 0.000323715353315892629 -0.000373797931366784408 0.000474735149205346429 -0.000620462923160480795 0.0008019470176010568 -0.00100763050558880241 0.0012242587423937773 -0.00143760444671135745 0.00163358485164961931 -0.00179904553508483667 0.00192273999864302214 -0.00199613698565934139 0.00201393108370888363 -0.00197453732615086863 0.00188017462496621601 -0.00173683589882892009 0.00155383993158385303 -0.00134339833613919546 0.00111969006640100233 -0.000898021861792566711 0.000693802895582407153 -0.000521451415147061725 0.000393460620889130031 -0.000319475280990855204 0.000305628182318204433 -0.00035398585438482788 0.000462449509504997414 -0.000624697261726536723 0.000830629806498964229 -0.00106696845123310791 0.00131808430223100126 -0.00156705540021362388 0.0017967751598609305 -0.00199113755689238336 0.0021361032376662481 -0.00222078893900451435 0.00223816501298737536 -0.00218569493865880538 0.00206555855995094184 -0.00188458904580310338 0.00165390732558040598 -0.00138823698768052173 0.00110497541323971438 -0.000823023495213667799 0.000561592912197900196 -0.000338804534440337313 0.00017050087627838717 -6.90690630648915782e-05 4.2529008939529156e-05 -9.38933246907719399e-05 0.000220865125287045272 -0.000415882968890834981 0.000666516090174193443 -0.000956269956464833593 0.00126556115154807802 -0.00157306787910335699 0.00185711629182253035 -0.00209717755977956166 0.00227529238813695134 -0.00237736926042747543 0.00239421768332964691 -0.00232227565890161247 0.00216401037953481423 -0.00192781610720255125 0.00162762600787852429 -0.00128203013052197168 0.000913117099558519163 -0.000545013068755595409 0.000202285101589816385 9.17616595409176394e-05 -0.000316706630690305468 0.000456456984326031323 -0.000500492956785919541 0.000444660340562730294 -0.0002916314312657875 5.08482703566182082e-05 0.000261964002217812686 -0.000625765149240259388 0.0010155069449110099 -0.00140378246659209061 0.00176267233724497485 -0.00206561757915099675 0.00228932009482940568 -0.00241538192609014324 0.00243170089546512758 -0.00233342243812229011 0.00212345832768764953 -0.0018124262750833231 0.00141811069229230702 -0.000964398418243000988 0.000479747548415287994 4.63530714139848143e-06 -0.000456908888136986491 0.000846756951237204181 -0.00114752653977315267 0.00133812278396319706 -0.00140461754828993812 0.00134134676684619092 -0.00115149343001350046 0.000847086736318197753 -0.00044834989969255723 -1.74786129602255702e-05 0.000517875135436357548 -0.00101713120254540157 0.00147876275019123704 -0.00186797193686399909 0.00215411163618373092 -0.00231287827978343685 0.00232812636500853709 -0.0021931879837525925 0.00191153727302703635 -0.00149680194099707786 0.000972054415599638011 ...(+9365 chars)]  InputProcessing=Columns as channels (frame based)
  Out : Outport  VectorParamsAs1DForOutWhenUnconnected=off
  wires:
  In/1 -> Generated Filter Block/1
  Generated Filter Block/1 -> Out/1
